simulink model "Phone_B"  (R2025a)
settings: Solver=FixedStepAuto  StartTime=0.0  StopTime=10.0  RelTol=1e-3
undefined symbols (not defined in the file): dspblkCoreblockFVToolHelper, gcbh
libraries: dspstat3 x2, androiduilib x1, androidaudiovideolib x1, androidcommunicationlib x1, dspadpt3 x1
settings Model: Creator=dell  LastModifiedBy=dell
settings OptimizationCC: DefaultParameterBehavior=Inlined  EnhancedBackFolding=on  PassReuseOutputArgsAs=Individual arguments  ZeroExternalMemoryAtStartup=off  ZeroInternalMemoryAtStartup=off  MaxStackSize=64  OptimizeBlockOrder=speed  DifferentSizesBufferReuse=on  OptimizationCustomize=off  EfficientTunableParamExpr=on
settings DebuggingCC: ParameterTunabilityLossMsg=error
settings HardwareCC: ProdBitPerLong=64.0  ProdLargestAtomicInteger=LongLong  ProdLargestAtomicFloat=Double  ProdLongLongMode=on  ProdHWDeviceType=ARM Compatible->ARM Cortex-A (64-bit)  UseEmbeddedCoderFeatures=off  UseSimulinkCoderFeatures=off
settings SFSimCC: MATLABDynamicMemAlloc=off
settings RTWCC: SystemTargetFile=ert.tlc  HardwareBoard=Android Device (64bit)  TLCOptions="-aInlineSetEventsForThisBaseRateFcn=TLC_FALSE -aSuppressMultiTaskScheduler=TLC_FALSE  -aRateBasedStepFcn=0"  TemplateMakefile=ert_default_tmf  RTWVerbose=off  Toolchain=Android SDK/NDK Tools  Description=Embedded Coder
settings CodeAppCC: ForceParamTrailComments=on  IgnoreCustomStorageClasses=off  OperatorAnnotations=on  SimulinkDataObjDesc=on  SFDataObjDesc=on  InsertBlockDesc=on
settings ERTTargetCC: ExtModeTransport=0.0  ExtModeStaticAlloc=off  ExtModeMexFile=ext_comm  ExtModeIntrfLevel=Level1  SupportNonInlinedSFcns=on

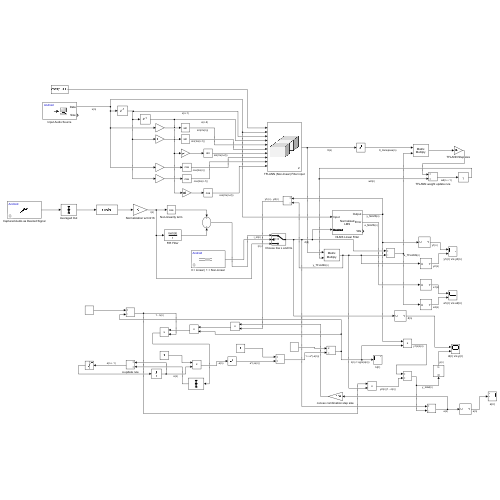
[thumbnail: Simulink's stored preview of the top-level diagram]
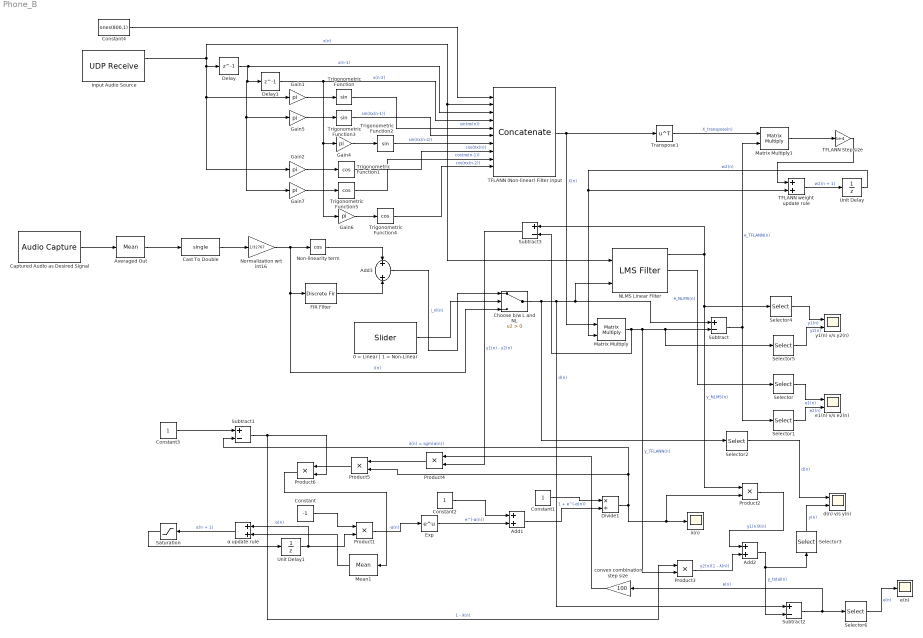
== system Phone_B ==
  0 = Linear | 1 = Non-Linear : androiduilib/Slider  Min=0  Value=1  Max=1  Resolution=1  SliderId=Phone_B/0_=_Linear_|_1_=_Non-Linear  SampleTime=0.1  BlockPlatform=Android
  Add1 : Sum
  Add2 : Sum
  Add3 : Sum
  Averaged Out : dspstat3/Mean  run=off  InputProcessing=Columns as channels (frame based)  reset_popup=None  directionMode=Each row  dimension=1  roiEnable=off  roiType=Rectangles  roiPortion=Entire ROI  roiOutput=Individual statistics for each ROI  roiFlag=off  roundingMode=Floor  overflowMode=off  outputDataTypeStr=Inherit: Same as accumulator  outputMin=[]  outputMax=[]  outputLastDataTypeStr=Inherit: Same as accumulator
  Captured Audio as Desired Signal : androidaudiovideolib/Audio Capture  SampleFreq=8000  FrameSize=800  SampleTime=0.1  SimulateUsing=Code generation  DeviceStr=0  QueueDuration=0  BlockPlatform=Android  AudioSamplingFreq=44100
  Cast To Double : DataTypeConversion  OutDataTypeStr=single  SaturateOnIntegerOverflow=off  RndMeth=Floor
  Choose b/w L and NL : Switch  Criteria=u2 > Threshold  SaturateOnIntegerOverflow=off  InputSameDT=off
  Constant : Constant  Value=-1  OutDataTypeStr=single
  Constant1 : Constant
  Constant2 : Constant
  Constant3 : Constant
  Constant4 : Constant  Value=ones(800,1)  VectorParams1D=off  OutDataTypeStr=single
  Delay : Delay  DelayLength=1  InputProcessing=Columns as channels (frame based)
  Delay1 : Delay  DelayLength=1  InputProcessing=Columns as channels (frame based)
  Divide1 : Product  Inputs=*/
  Exp : Math
  FIR Filter : DiscreteFir  LoadFcn=dspblkCoreblockFVToolHelper(gcbh,'load');  Coefficients=[.3 0.9 .4 -.3 -.7]  InputProcessing=Columns as channels (frame based)
      settings: CopyFcn=dspblkCoreblockFVToolHelper(gcbh,'copy');  DeleteFcn=dspblkCoreblockFVToolHelper(gcbh,'close');  ModelCloseFcn=dspblkCoreblockFVToolHelper(gcbh,'close');  PreSaveFcn=dspblkCoreblockFVToolHelper(gcbh,'presave');  PostSaveFcn=dspblkCoreblockFVToolHelper(gcbh,'postsave');  CloseFcn=dspblkCoreblockFVToolHelper(gcbh,'close');
  Gain{1..2,4..7} (6 alike) : Gain  Gain=pi
  Input Audio Source : androidcommunicationlib/UDP Receive  localURL='0.0.0.0'  localPort=25000  remoteURL='0.0.0.0'  remotePort=-1  recvBufferSize=8192  signalDatatype=single  dims=800  isVarSize=off  showBlockingTime=off  blockingTime=0  sampletime=0.1  blockPlatform=Android
  Matrix Multiply : Product  Multiplication=Matrix(*)
  Matrix Multiply1 : Product  Multiplication=Matrix(*)
  Mean1 : dspstat3/Mean  run=off  InputProcessing=Columns as channels (frame based)  reset_popup=None  directionMode=Each column  dimension=1  roiEnable=off  roiType=Rectangles  roiPortion=Entire ROI  roiOutput=Individual statistics for each ROI  roiFlag=off  roundingMode=Floor  overflowMode=off  outputDataTypeStr=Inherit: Same as accumulator  outputMin=[]  outputMax=[]  outputLastDataTypeStr=Inherit: Same as accumulator
  NLMS Linear Filter : dspadpt3/LMS Filter  Algo=Normalized LMS  L=8  stepflag=Dialog  mu=1  leakage=1.0  ic=0  Adapt=off  resetflag=None  weights=on  addnparflag=off  roundingMode=Floor  overflowMode=off
  Non-linearity term : Trigonometry  Operator=cos
  Normalization wrt int16 : Gain  Gain=1/32767
  Product{1..6} (6 alike) : Product
  Saturation : Saturate  UpperLimit=4  LowerLimit=-4
  Selector{,1..6} (7 alike) : Selector  InputPortWidth=800  IndexOptions=Index vector (dialog)  Indices=[1]  OutputSizes=1
  Subtract{,1..3} (4 alike) : Sum  Inputs=+-
  TFLANN (Non-linear) Filter input : Concatenate  NumInputs=10  Mode=Multidimensional array  ConcatenateDimension=2
  TFLANN Step size : Gain  Gain=1e-4
  TFLANN weight update rule : Sum
  Transpose1 : Math  Operator=transpose
  Trigonometric Function : Trigonometry  ApproximationMethod=Lookup
  Trigonometric Function1 : Trigonometry  Operator=cos  ApproximationMethod=Lookup
  Trigonometric Function2 : Trigonometry  ApproximationMethod=Lookup
  Trigonometric Function3 : Trigonometry  ApproximationMethod=Lookup
  Trigonometric Function4 : Trigonometry  Operator=cos  ApproximationMethod=Lookup
  Trigonometric Function5 : Trigonometry  Operator=cos  ApproximationMethod=Lookup
  Unit Delay : UnitDelay  InitialCondition=zeros(10,1)  SampleTime=-1  HasFrameUpgradeWarning=on
  Unit Delay1 : UnitDelay  SampleTime=-1  HasFrameUpgradeWarning=on
  convex combination step size : Gain  Gain=100
  d(n) v/s y(n) : Scope  NumInputPorts=2
      settings: ActiveDisplayYMinimum=-1  ActiveDisplayYMaximum=1  DataLoggingVariableName=ScopeData2
  e(n) : Scope
      settings: ActiveDisplayYMinimum=-1  ActiveDisplayYMaximum=1  DataLoggingVariableName=ScopeData4
  e1(n) v/s e2(n) : Scope  NumInputPorts=2
      settings: ActiveDisplayYMinimum=-1  ActiveDisplayYMaximum=1
  y1(n) v/s y2(n) : Scope  NumInputPorts=2
      settings: ActiveDisplayYMinimum=-1  ActiveDisplayYMaximum=1  DataLoggingVariableName=ScopeData3
  α update rule : Sum
  λ(n) : Scope
      settings: ActiveDisplayYMinimum=0  ActiveDisplayYMaximum=1
  wires:
  Add2/1 -> Selector3/1, Subtract2/2  "y_total(n)"
  Add3/1 -> Choose b/w L and NL/1  "i_nl(n)"
  α update rule/1 -> Saturation/1  "α(n + 1)"
  0 = Linear | 1 = Non-Linear/1 -> Choose b/w L and NL/2
  Saturation/1 -> Unit Delay1/1
  Captured Audio as Desired Signal/1 -> Averaged Out/1
  Unit Delay/1 -> Matrix Multiply/2, TFLANN weight update rule/2  "w2(n)"
  Trigonometric Function3/1 -> TFLANN (Non-linear) Filter input/6  "sin(πx(n-1))"
  Input Audio Source/1 -> Gain2/1, Gain1/1, Delay/1, TFLANN (Non-linear) Filter input/2, NLMS Linear Filter/1  "x(n)"
  Averaged Out/1 -> Cast To Double/1
  Delay/1 -> TFLANN (Non-linear) Filter input/3, Delay1/1, Gain7/1, Gain5/1  "x(n-1)"
  Constant1/1 -> Divide1/1
  Constant3/1 -> Subtract1/1
  Gain1/1 -> Trigonometric Function/1
  Gain2/1 -> Trigonometric Function1/1
  Cast To Double/1 -> Normalization wrt int16/1
  Subtract2/1 -> convex combination step size/1, Selector6/1  "e(n)"
  Subtract/1 -> Selector1/1, Matrix Multiply1/2  "e_TFLANN(n)"
  Subtract3/1 -> Product4/2  "y1(n) - y2(n)"
  Subtract1/1 -> Product6/2, Product3/1  "1 - λ(n)"
  Product5/1 -> Product6/1
  Product6/1 -> Mean1/1
  Trigonometric Function/1 -> TFLANN (Non-linear) Filter input/5  "sin(πx(n))"
  Gain5/1 -> Trigonometric Function3/1
  Gain7/1 -> Trigonometric Function5/1
  Gain4/1 -> Trigonometric Function2/1
  Normalization wrt int16/1 -> Choose b/w L and NL/3, FIR Filter/1, Non-linearity term/1  "i(n)"
  Constant2/1 -> Add1/1
  Constant4/1 -> TFLANN (Non-linear) Filter input/1
  Constant/1 -> Product1/1
  Unit Delay1/1 -> α update rule/1, Product1/2  "α(n)"
  Mean1/1 -> α update rule/2
  Trigonometric Function5/1 -> TFLANN (Non-linear) Filter input/9  "cos(πx(n-1))"
  Gain6/1 -> Trigonometric Function4/1
  Selector3/1 -> d(n) v/s y(n)/2  "y(n)"
  Non-linearity term/1 -> Add3/1
  Divide1/1 -> λ(n)/1, Product2/2, Subtract1/2, Product5/2  "λ(n) = sgm(α(n))"
  FIR Filter/1 -> Add3/2
  Product3/1 -> Add2/2  "y2(n)(1 - λ(n))"
  Product2/1 -> Add2/1  "y1(n)λ(n)"
  Product4/1 -> Product5/1
  Product1/1 -> Exp/1  "-α(n)"
  Trigonometric Function2/1 -> TFLANN (Non-linear) Filter input/7  "sin(πx(n-2))"
  Trigonometric Function1/1 -> TFLANN (Non-linear) Filter input/8  "cos(πx(n))"
  Trigonometric Function4/1 -> TFLANN (Non-linear) Filter input/10  "cos(πx(n-2))"
  convex combination step size/1 -> Product4/1
  Exp/1 -> Add1/2  "e^(-α(n))"
  TFLANN (Non-linear) Filter input/1 -> Transpose1/1, Matrix Multiply/1  "X(n)"
  Choose b/w L and NL/1 -> Subtract2/1, Subtract/1, NLMS Linear Filter/2, Selector2/1  "d(n)"
  TFLANN weight update rule/1 -> Unit Delay/1  "w2(n + 1)"
  Add1/1 -> Divide1/2  "1 + e^(-α(n))"
  Transpose1/1 -> Matrix Multiply1/1  "X_transpose(n)"
  NLMS Linear Filter/1 -> Product2/1, Selector4/1, Subtract3/1  "y_NLMS(n)"
  NLMS Linear Filter/2 -> Selector/1  "e_NLMS(n)"
  Matrix Multiply1/1 -> TFLANN Step size/1
  Matrix Multiply/1 -> Selector5/1, Subtract/2, Product3/2, Subtract3/2  "y_TFLANN(n)"
  Selector4/1 -> y1(n) v/s y2(n)/1  "y1(n)"
  Selector5/1 -> y1(n) v/s y2(n)/2  "y2(n)"
  Selector/1 -> e1(n) v/s e2(n)/1  "e1(n)"
  Selector1/1 -> e1(n) v/s e2(n)/2  "e2(n)"
  Selector6/1 -> e(n)/1  "e(n)"
  Selector2/1 -> d(n) v/s y(n)/1  "d(n)"
  TFLANN Step size/1 -> TFLANN weight update rule/1
  Delay1/1 -> TFLANN (Non-linear) Filter input/4, Gain6/1, Gain4/1  "x(n-2)"
